simulink model "Cruise_control_V5"  (R2017a)
settings: Solver=VariableStepAuto  StartTime=0.0  StopTime=300  RelTol=1e-3
values from neighbouring files (symbols this model uses):
  DENSITY = 1.164    [parameters.m]
  DRAG_COEFF = 0.2    [parameters.m]
  EMOTOR_EFF = 0.945    [parameters.m]
  energyTotal_noDrag = energyTotal_noDrag/(3600*EMOTOR_EFF)    [parameters.m]
  FRICTION_COEFF = 0.02    [parameters.m]
  HorizontalGravityForce = data(:,4)    [parameters.m]
  MASS = 250    [parameters.m]
  MAX_SPEED = 100/1.60934    (= 62.137273665)    [parameters.m]
  mult_vel_ToPower = mult_vel_ToPower*1.60934/(3.6*EMOTOR_EFF)    [parameters.m]
  mult_velcubed_ToPower = DENSITY*DRAG_COEFF*1.60934^3/(2*3.6^3*EMOTOR_EFF)    (= 0.0110041648249)    [parameters.m]
  mult_velsq_ToDragEnergy = DENSITY*DRAG_COEFF*1000*1.60934^3/(2*3.6^2)    (= 37.4361687342)    [parameters.m]
  NetDistancemiles = data(:,2)    [parameters.m]
  total_distmiles = NetDistancemiles(len)+Distancemiles(len)    [parameters.m]
  WARNING_LIGHT = 0.15    [parameters.m]
undefined symbols (not defined in the file or in its folder): magnitude, sigbuilder_block
libraries: simulink x2, commutil2 x1
settings Model: PauseTimes=15  Creator=marty  LastModifiedBy=marty
settings OptimizationCC: DefaultParameterBehavior=Inlined  UseDivisionForNetSlopeComputation=on  UseFloatMulNetSlope=on  InlineInvariantSignals=on  PassReuseOutputArgsAs=Individual arguments  ZeroExternalMemoryAtStartup=off  ZeroInternalMemoryAtStartup=off  NoFixptDivByZeroProtection=on  EfficientFloat2IntCast=on  LifeSpan=1
settings DebuggingCC: ParameterTunabilityLossMsg=error
settings HardwareCC: ProdBitPerInt=16  ProdBitPerPointer=8  ProdBitPerSizeT=24  ProdBitPerPtrDiffT=24  ProdLargestAtomicFloat=None  ProdWordSize=8  ProdHWDeviceType=Microchip->PIC18
settings SFSimCC: MATLABDynamicMemAlloc=off
settings RTWCC: SystemTargetFile=ert.tlc  TemplateMakefile=ert_default_tmf  Description=Embedded Coder  GenerateReport=on  IncludeHyperlinkInReport=on  LaunchReport=on  GenerateTraceInfo=on  GenerateTraceReport=on  GenerateTraceReportSl=on  GenerateTraceReportSf=on  GenerateTraceReportEml=on  GenerateCodeMetricsReport=on
settings CodeAppCC: ForceParamTrailComments=on  IgnoreCustomStorageClasses=off  OperatorAnnotations=on  SimulinkDataObjDesc=on  SFDataObjDesc=on  MATLABFcnDesc=on  CustomSymbolStrGlobalVar=rt$N$M  CustomSymbolStrType=$N$M  CustomSymbolStrFcn=$N$M$F  CustomSymbolStrMacro=$N$M  InsertBlockDesc=on  MATLABSourceComments=on
settings ERTTargetCC: TargetLangStandard=C99 (ISO)  GenerateSampleERTMain=on  IncludeMdlTerminateFcn=off  CombineSignalStateStructs=on  SupportContinuousTime=on  SupportNonInlinedSFcns=on  SupportVariableSizeSignals=on  InlinedParameterPlacement=NonHierarchical  ERTCustomFileTemplate=example_file_process.tlc  ERTFilePackagingFormat=CompactWithDataFile

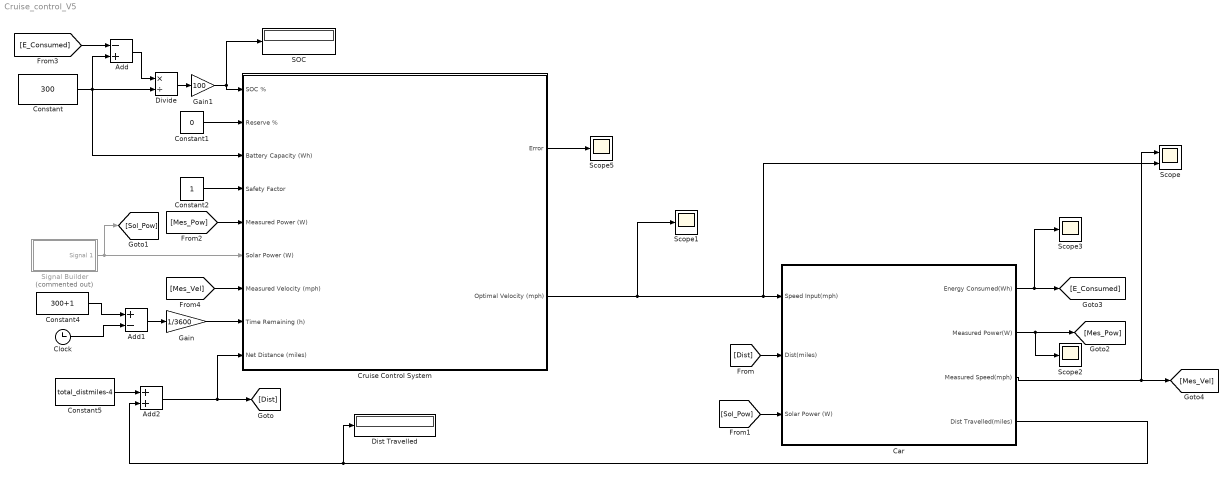
== system Cruise_control_V5 ==
  Add : Sum  Inputs=-+
  Add1 : Sum  Inputs=+-
  Add2 : Sum
  Car : Subsystem
  Clock : Clock
  Constant : Constant  Value=300
  Constant1 : Constant  Value=0
  Constant2 : Constant
  Constant4 : Constant  Value=300+1
  Constant5 : Constant  Value=total_distmiles-4
  Cruise Control System : Subsystem
  Dist Travelled : Display
  Divide : Product  Inputs=*/
  Gain : Gain  Gain=1/3600
  Gain1 : Gain  Gain=100
  SOC : Display
  Scope : Scope  NumInputPorts=2
  Scope{1..3,5} (4 alike) : Scope
  Signal Builder : Subsystem  Tag=STV Subsys  Commented=on  LoadFcn=sigbuilder_block('load');  StartFcn=sigbuilder_block('start');  StopFcn=sigbuilder_block('stop');  ClipboardFcn=sigbuilder_block('clipboard');  mask(Sigbuilder block){tuvar=[0:10]}
      mask help: Simulink:masks:SigbuilderBlock_MD
      mask init:
      | if ~strcmp(get_param(bdroot(gcbh),'SimulationStatus'),'stopped') tuvar = sigbuilder_block('maskInit'); end
      settings: CopyFcn=sigbuilder_block('copy');  DeleteFcn=sigbuilder_block('delete');  ModelCloseFcn=sigbuilder_block('modelClose');  PreSaveFcn=sigbuilder_block('preSave');  PauseFcn=sigbuilder_block('pause');  ContinueFcn=sigbuilder_block('continue');  NameChangeFcn=sigbuilder_block('namechange');  OpenFcn=sigbuilder_block('open',[281.4 73.8 550.8 400.2 ]);  CloseFcn=sigbuilder_block('close');
      mask Display: plot(0, 0, 100, 100,[2, 2, 32, 32, 2], [68, 8, 8, 68, 68],[32, 2], [38, 38], [32, 19, 2],[53, 60, 44], [32, 17, 17, 2],[16, 16, 31, 31]);txt = getActiveGroup(gcbh);text(2, 100, txt,'verticalAlignment', 'top');
  wires:
  Add/1 -> Divide/1
  Constant/1 -> Cruise Control System/3(Battery Capacity (Wh)), Divide/2, Add/2
  Constant1/1 -> Cruise Control System/2(Reserve %)
  Constant2/1 -> Cruise Control System/4(Safety Factor)
  Signal Builder/1(Signal 1) -> [Sol_Pow], Cruise Control System/6(Solar Power (W))
  Constant4/1 -> Add1/1
  Clock/1 -> Add1/2
  Add1/1 -> Gain/1
  Constant5/1 -> Add2/1
  Car/4(Dist Travelled(miles)) -> Dist Travelled/1, Add2/2
  Add2/1 -> [Dist], Cruise Control System/9(Net Distance (miles))
  Divide/1 -> Gain1/1
  Gain1/1 -> SOC/1, Cruise Control System/1(SOC %)
  Gain/1 -> Cruise Control System/8(Time Remaining (h))
  [Dist] -> Car/2(Dist(miles))
  Cruise Control System/1(Error) -> Scope5/1
  [Sol_Pow] -> Car/3(Solar Power (W))
  Car/2(Measured Power(W)) -> Scope2/1, [Mes_Pow]
  [Mes_Pow] -> Cruise Control System/5(Measured Power (W))
  Car/1(Energy Consumed(Wh)) -> Scope3/1, [E_Consumed]
  [E_Consumed] -> Add/1
  Car/3(Measured Speed(mph)) -> Scope/1, [Mes_Vel]
  [Mes_Vel] -> Cruise Control System/7(Measured Velocity (mph))
  Cruise Control System/2(Optimal Velocity (mph)) -> Scope/2, Car/1(Speed Input(mph)), Scope1/1

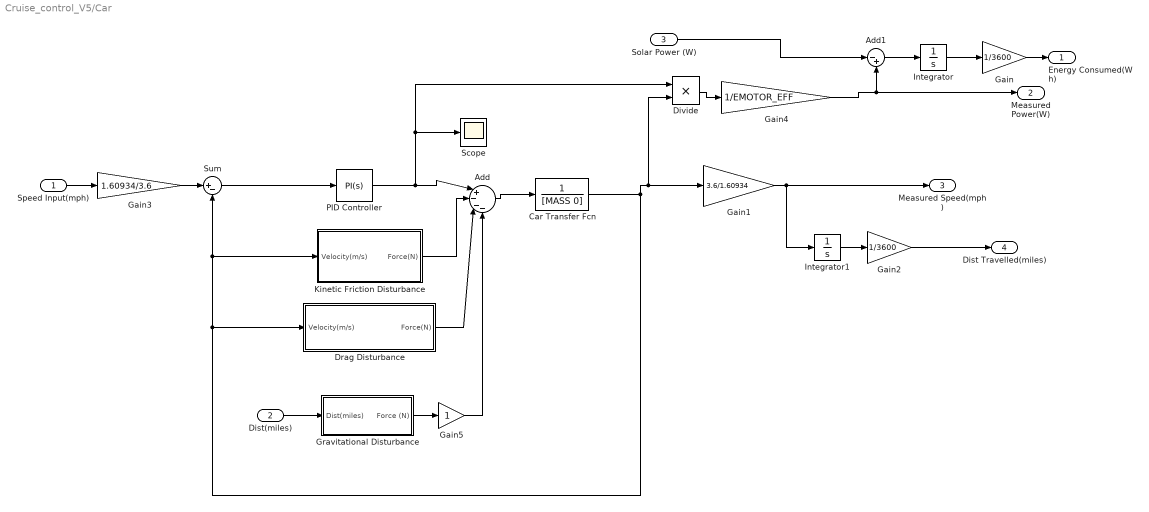
== system Cruise_control_V5/Car ==
  Speed Input(mph) : Inport
  Dist(miles) : Inport  Port=2
  Solar Power (W) : Inport  Port=3
  Add : Sum  Inputs=|+---
  Add1 : Sum  Inputs=|-+
  Car Transfer Fcn : TransferFcn  Denominator=[MASS 0]
  Divide : Product  Inputs=**
  Drag Disturbance : Subsystem
  Gain : Gain  Gain=1/3600
  Gain1 : Gain  Gain=3.6/1.60934
  Gain2 : Gain  Gain=1/3600
  Gain3 : Gain  Gain=1.60934/3.6
  Gain4 : Gain  Gain=1/EMOTOR_EFF
  Gain5 : Gain
  Gravitational Disturbance : Subsystem
  Integrator : Integrator
  Integrator1 : Integrator
  Kinetic Friction Disturbance : Subsystem
  PID Controller : simulink/Continuous/PID Controller  Controller=PI  TimeDomain=Continuous-time  SampleTime=-1  IntegratorMethod=Forward Euler  FilterMethod=Forward Euler  Form=Parallel  UseFilter=on  ControllerParametersSource=internal  P=200  I=19.1491594951774  D=-103.133475492692  N=0.374096308615762  InitialConditionSource=internal  InitialConditionForIntegrator=0  InitialConditionForFilter=0  ExternalReset=none  LimitOutput=off  UpperSaturationLimit=inf  LowerSaturationLimit=-inf  LinearizeAsGain=on  AntiWindupMode=none  Kb=1  TrackingMode=off  Kt=1  PParamMin=[]  PParamMax=[]  IParamMin=[]  IParamMax=[]  DParamMin=[]  DParamMax=[]  NParamMin=[]  NParamMax=[]  KbParamMin=[]  KbParamMax=[]  KtParamMin=[]  KtParamMax=[]  POutMin=[]  POutMax=[]  IOutMin=[]  IOutMax=[]  DOutMin=[]  DOutMax=[]  NOutMin=[]  NOutMax=[]  KbOutMin=[]  KbOutMax=[]  KtOutMin=[]  KtOutMax=[]  IntegratorOutMin=[]  IntegratorOutMax=[]  FilterOutMin=[]  FilterOutMax=[]  SumOutMin=[]  SumOutMax=[]  SumI1OutMin=[]  SumI1OutMax=[]  SumI2OutMin=[]  SumI2OutMax=[]  SumI3OutMin=[]  SumI3OutMax=[]  SumDOutMin=[]  SumDOutMax=[]  SaturationOutMin=[]  SaturationOutMax=[]  IntegratorContinuousStateAttributes=''  IntegratorStateMustResolveToSignalObject=off  IntegratorRTWStateStorageClass=Auto  FilterContinuousStateAttributes=''  FilterStateMustResolveToSignalObject=off  FilterRTWStateStorageClass=Auto  DifferentiatorICPrevScaledInput=0  DifferentiatorOutMin=[]  DifferentiatorOutMax=[]  InitialConditionSetting=State (most efficient)
  Scope : Scope
  Sum : Sum  Inputs=|+-
  Energy Consumed(Wh) : Outport
  Measured Power(W) : Outport  Port=2
  Measured Speed(mph) : Outport  Port=3
  Dist Travelled(miles) : Outport  Port=4
  wires:
  Sum/1 -> PID Controller/1
  Car Transfer Fcn/1 -> Gain1/1, Divide/2, Sum/2, Kinetic Friction Disturbance/1(Velocity(m/s)), Drag Disturbance/1(Velocity(m/s))
  Divide/1 -> Gain4/1
  Integrator/1 -> Gain/1
  Gain/1 -> Energy Consumed(Wh)/1
  Gain3/1 -> Sum/1
  Gain1/1 -> Integrator1/1, Measured Speed(mph)/1
  Integrator1/1 -> Gain2/1
  Gain2/1 -> Dist Travelled(miles)/1
  Speed Input(mph)/1 -> Gain3/1
  Add/1 -> Car Transfer Fcn/1
  Kinetic Friction Disturbance/1(Force(N)) -> Add/2
  Drag Disturbance/1(Force(N)) -> Add/3
  Dist(miles)/1 -> Gravitational Disturbance/1(Dist(miles))
  Gain4/1 -> Add1/2, Measured Power(W)/1
  Add1/1 -> Integrator/1
  Solar Power (W)/1 -> Add1/1
  PID Controller/1 -> Scope/1, Divide/1, Add/1
  Gravitational Disturbance/1(Force (N)) -> Gain5/1
  Gain5/1 -> Add/4

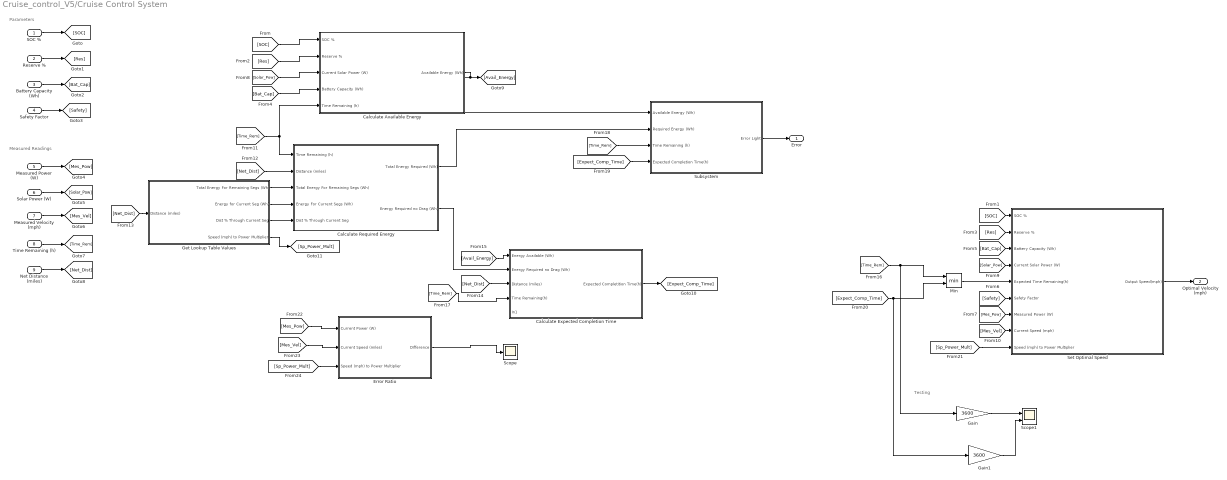
== system Cruise_control_V5/Cruise Control System ==
  note: Testing
  note: Measured Readings
  note: Parameters
  SOC % : Inport
  Reserve % : Inport  Port=2
  Battery Capacity (Wh) : Inport  Port=3
  Safety Factor : Inport  Port=4
  Measured Power (W) : Inport  Port=5
  Solar Power (W) : Inport  Port=6
  Measured Velocity (mph) : Inport  Port=7
  Time Remaining (h) : Inport  Port=8
  Net Distance (miles) : Inport  Port=9
  Calculate Available Energy : Subsystem
  Calculate Expected Completion Time : Subsystem
  Calculate Required Energy : Subsystem
  Error Ratio : Subsystem
  Gain : Gain  Gain=3600
  Gain1 : Gain  Gain=3600
  Get Lookup Table Values : Subsystem
  Min : MinMax  Inputs=2
  Scope : Scope
  Scope1 : Scope  NumInputPorts=2
  Set Optimal Speed : Subsystem
  Subsystem : Subsystem
  Error : Outport
  Optimal Velocity (mph) : Outport  Port=2
  wires:
  Time Remaining (h)/1 -> [Time_Rem]
  Solar Power (W)/1 -> [Solar_Pow]
  Measured Velocity (mph)/1 -> [Mes_Vel]
  [Solar_Pow] -> Set Optimal Speed/4(Current Solar Power (W))
  [Solar_Pow] -> Calculate Available Energy/3(Current Solar Power (W))
  [SOC] -> Set Optimal Speed/1(SOC %)
  Set Optimal Speed/1(Output Speed(mph)) -> Optimal Velocity (mph)/1
  [Res] -> Calculate Available Energy/2(Reserve %)
  Battery Capacity (Wh)/1 -> [Bat_Cap]
  [Bat_Cap] -> Set Optimal Speed/3(Battery Capacity (Wh))
  Net Distance (miles)/1 -> [Net_Dist]
  Get Lookup Table Values/3(Dist % Through Current Seg) -> Calculate Required Energy/5(Dist % Through Current Seg)
  [Mes_Pow] -> Set Optimal Speed/7(Measured Power (W))
  [Bat_Cap] -> Calculate Available Energy/4(Battery Capacity (Wh))
  Measured Power (W)/1 -> [Mes_Pow]
  Get Lookup Table Values/2(Energy for Current Seg (Wh)) -> Calculate Required Energy/4(Energy For Current Segs (Wh))
  Get Lookup Table Values/1(Total Energy For Remaining Segs (Wh)) -> Calculate Required Energy/3(Total Energy For Remaining Segs (Wh))
  [Res] -> Set Optimal Speed/2(Reserve %)
  Reserve %/1 -> [Res]
  [SOC] -> Calculate Available Energy/1(SOC %)
  SOC %/1 -> [SOC]
  [Safety] -> Set Optimal Speed/6(Safety Factor)
  [Net_Dist] -> Calculate Required Energy/2("Distance (miles) ")
  [Mes_Vel] -> Set Optimal Speed/8(Current Speed (mph))
  Safety Factor/1 -> [Safety]
  [Time_Rem] -> Calculate Required Energy/1(Time Remaining (h)), Calculate Available Energy/5(Time Remaining (h))
  Calculate Required Energy/2(Energy Required no Drag (Wh)) -> Calculate Expected Completion Time/2(Energy Required no Drag (Wh))
  [Net_Dist] -> Get Lookup Table Values/1(Distance (miles))
  Calculate Required Energy/1(Total Energy Required (Wh)) -> Subsystem/2(Required Energy (Wh))
  Calculate Available Energy/1(Available Energy (Wh)) -> Subsystem/1(Available Energy (Wh)), [Avail_Energy]
  [Net_Dist] -> Calculate Expected Completion Time/3("Distance (miles) ")
  Min/1 -> Set Optimal Speed/5(Expected Time Remaining(h))
  [Time_Rem] -> Calculate Expected Completion Time/4(Time Remaining(h))
  Gain/1 -> Scope1/1
  Gain1/1 -> Scope1/2
  [Avail_Energy] -> Calculate Expected Completion Time/1(Energy Available (Wh))
  [Time_Rem] -> Min/1, Gain/1
  [Time_Rem] -> Subsystem/3(Time Remaining (h))
  Calculate Expected Completion Time/1("Expected Completition Time(h) ") -> [Expect_Comp_Time]
  [Expect_Comp_Time] -> Subsystem/4(Expected Completion Time(h))
  [Expect_Comp_Time] -> Min/2, Gain1/1
  Get Lookup Table Values/4(Speed (mph) to Power Multiplier) -> [Sp_Power_Mult]
  [Sp_Power_Mult] -> Set Optimal Speed/9(Speed (mph) to Power Multiplier)
  Subsystem/1("Error Light ") -> Error/1
  Error Ratio/1(Difference) -> Scope/1
  [Mes_Pow] -> Error Ratio/1(Current Power (W))
  [Mes_Vel] -> Error Ratio/2(Current Speed (miles))
  [Sp_Power_Mult] -> Error Ratio/3("Speed (mph) to Power Multiplier ")

== system Cruise_control_V5/Signal Builder ==
  Demux : Demux  Tag=STV Demux  Outputs=1
  FromWs : FromWorkspace  Tag=STV FromWs  VariableName=tuvar  SampleTime=0
      SigBuilderData=|
      | common.afterFinalStr = 'Extrapolate'
      | common.sampleTime = 0
      | dataSet.timeRange = [0 120]
      | dataSet.name = 'Group 1'
      | sbobj.Groups.Name = 'Group 1'
      | sbobj.Groups.Signals.Name = 'Signal 1'
      | sbobj.Groups.Signals.XData = [0 4 6 40 40 120]
      | sbobj.Groups.Signals.YData = [0 0 0 0 750 750]
      | sbobj.Groups.TimeRange = [0 120]
  Signal 1 : Outport  Tag=STV Outport
  wires:
  Demux/1 -> Signal 1/1
  FromWs/1 -> Demux/1

== system Cruise_control_V5/Car/Drag Disturbance ==
  Velocity(m/s) : Inport
  Display : Display
  Gain5 : Gain  Gain=DENSITY*DRAG_COEFF/2
  Math Function : Math  Operator=magnitude^2  SaturateOnIntegerOverflow=on
  Force(N) : Outport
  wires:
  Gain5/1 -> Force(N)/1
  Math Function/1 -> Gain5/1
  Velocity(m/s)/1 -> Display/1, Math Function/1

== system Cruise_control_V5/Car/Gravitational Disturbance ==
  Dist(miles) : Inport
  Direct Lookup Table (n-D) : LookupNDDirect  NumberOfTableDimensions=1  Table=[HorizontalGravityForce']
  Prelookup : PreLookup  BreakpointsData=[NetDistancemiles;total_distmiles]
  Force (N) : Outport
  wires:
  Prelookup/1 -> Direct Lookup Table (n-D)/1
  Dist(miles)/1 -> Prelookup/1
  Direct Lookup Table (n-D)/1 -> Force (N)/1

== system Cruise_control_V5/Car/Kinetic Friction Disturbance ==
  Velocity(m/s) : Inport
  Constant : Constant  Value=MASS*9.8*FRICTION_COEFF
  Constant1 : Constant  Value=0
  Switch : Switch  Criteria=u2 > Threshold
  Force(N) : Outport
  wires:
  Switch/1 -> Force(N)/1
  Constant1/1 -> Switch/3
  Velocity(m/s)/1 -> Switch/2
  Constant/1 -> Switch/1

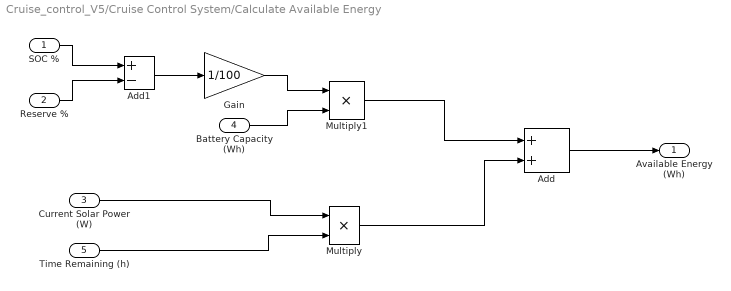
== system Cruise_control_V5/Cruise Control System/Calculate Available Energy ==
  SOC % : Inport
  Reserve % : Inport  Port=2
  Current Solar Power (W) : Inport  Port=3
  Battery Capacity (Wh) : Inport  Port=4
  Time Remaining (h) : Inport  Port=5
  Add : Sum
  Add1 : Sum  Inputs=+-
  Gain : Gain  Gain=1/100
  Multiply : Product  Inputs=**
  Multiply1 : Product  Inputs=**
  Available Energy (Wh) : Outport
  wires:
  SOC %/1 -> Add1/1
  Multiply/1 -> Add/2
  Gain/1 -> Multiply1/1
  Add1/1 -> Gain/1
  Reserve %/1 -> Add1/2
  Multiply1/1 -> Add/1
  Battery Capacity (Wh)/1 -> Multiply1/2
  Current Solar Power (W)/1 -> Multiply/1
  Time Remaining (h)/1 -> Multiply/2
  Add/1 -> Available Energy (Wh)/1

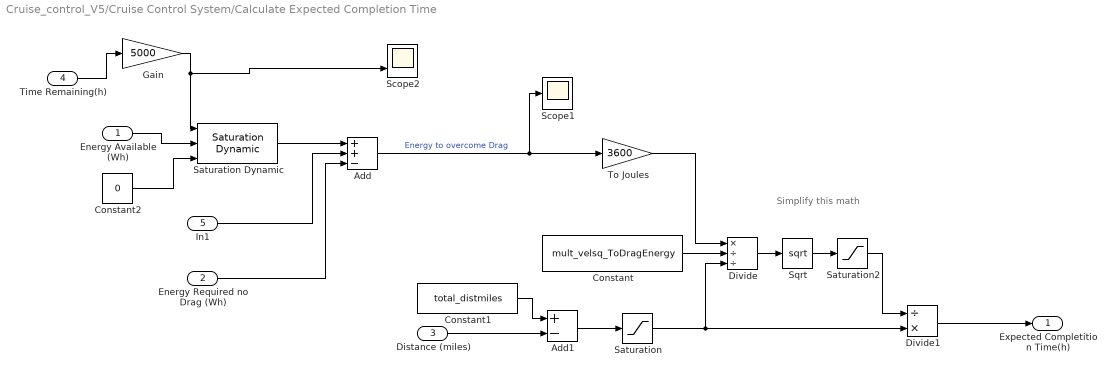
== system Cruise_control_V5/Cruise Control System/Calculate Expected Completion Time ==
  note: Simplify this math
  Energy Available (Wh) : Inport
  Energy Required no Drag (Wh) : Inport  Port=2
  "Distance (miles) " : Inport  Port=3
  Time Remaining(h) : Inport  Port=4
  In1 : Inport  Port=5
  Add : Sum  Inputs=++-
  Add1 : Sum  Inputs=+-
  Constant : Constant  Value=mult_velsq_ToDragEnergy  SampleTime=-1
  Constant1 : Constant  Value=total_distmiles
  Constant2 : Constant  Value=0
  Divide : Product  Inputs=*//
  Divide1 : Product  Inputs=/*
  Gain : Gain  Gain=5000
  Saturation : Saturate  UpperLimit=inf  LowerLimit=0
  Saturation Dynamic : simulink/Discontinuities/Saturation Dynamic  OutMin=[]  OutMax=[]  OutDataTypeStr=Inherit: Same as second input  OutDataType=fixdt(1, 16)  OutScaling=2^-10  DoSatur=off
  Saturation2 : Saturate  UpperLimit=MAX_SPEED  LowerLimit=0
  Scope1 : Scope
  Scope2 : Scope  NumInputPorts=2
  Sqrt : Sqrt  SaturateOnIntegerOverflow=on
  To Joules : Gain  Gain=3600
  "Expected Completition Time(h) " : Outport
  wires:
  Add/1 -> Scope1/1, To Joules/1  "Energy to overcome Drag"
  To Joules/1 -> Divide/1
  Sqrt/1 -> Saturation2/1
  Divide1/1 -> "Expected Completition Time(h) "/1
  Constant1/1 -> Add1/1
  "Distance (miles) "/1 -> Add1/2
  Constant/1 -> Divide/2
  Add1/1 -> Saturation/1
  Saturation/1 -> Divide1/2, Divide/3
  Time Remaining(h)/1 -> Gain/1
  Constant2/1 -> Saturation Dynamic/3
  Gain/1 -> Saturation Dynamic/1, Scope2/2
  Saturation Dynamic/1 -> Add/1
  Energy Available (Wh)/1 -> Saturation Dynamic/2
  Divide/1 -> Sqrt/1
  Saturation2/1 -> Divide1/1
  In1/1 -> Add/2
  Energy Required no Drag (Wh)/1 -> Add/3

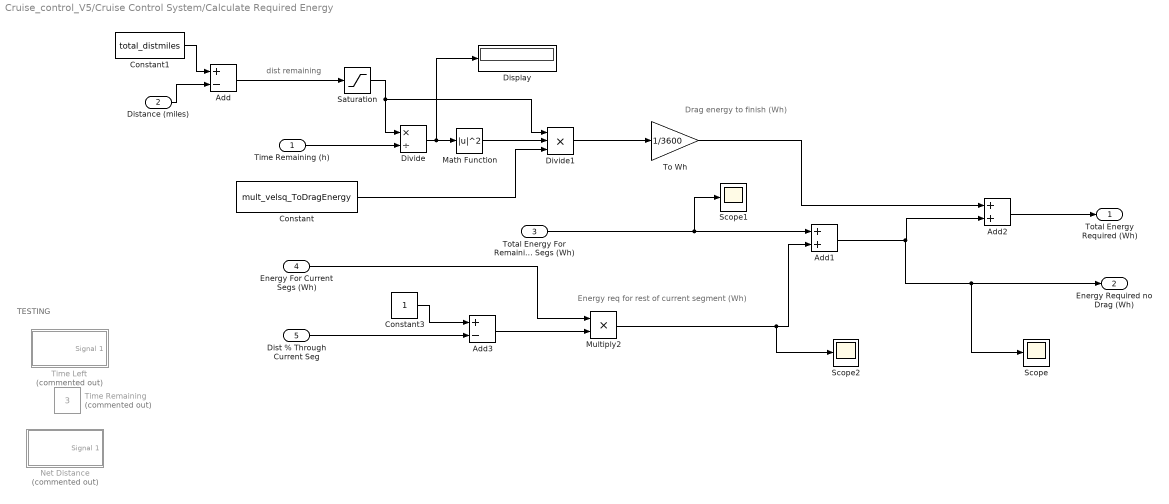
== system Cruise_control_V5/Cruise Control System/Calculate Required Energy ==
  note: TESTING
  note: Drag energy to finish (Wh)
  note: dist remaining
  note: Energy req for rest of current segment (Wh)
  Time Remaining (h) : Inport
  "Distance (miles) " : Inport  Port=2
  Total Energy For Remaining Segs (Wh) : Inport  Port=3
  Energy For Current Segs (Wh) : Inport  Port=4
  Dist % Through Current Seg : Inport  Port=5
  Add : Sum  Inputs=+-
  Add1 : Sum
  Add2 : Sum
  Add3 : Sum  Inputs=+-
  Constant : Constant  Value=mult_velsq_ToDragEnergy  SampleTime=-1
  Constant1 : Constant  Value=total_distmiles
  Constant3 : Constant
  Display : Display
  Divide : Product  Inputs=*/
  Divide1 : Product  Inputs=***
  Math Function : Math  Operator=magnitude^2  SaturateOnIntegerOverflow=on
  Multiply2 : Product  Inputs=**
  Net Distance : Subsystem  Tag=STV Subsys  Commented=on  LoadFcn=sigbuilder_block('load');  StartFcn=sigbuilder_block('start');  StopFcn=sigbuilder_block('stop');  ClipboardFcn=sigbuilder_block('clipboard');  mask(Sigbuilder block){tuvar=[0:10]}
      mask help: Simulink:masks:SigbuilderBlock_MD
      mask init:
      | if ~strcmp(get_param(bdroot(gcbh),'SimulationStatus'),'stopped') tuvar = sigbuilder_block('maskInit'); end
      settings: CopyFcn=sigbuilder_block('copy');  DeleteFcn=sigbuilder_block('delete');  ModelCloseFcn=sigbuilder_block('modelClose');  PreSaveFcn=sigbuilder_block('preSave');  PauseFcn=sigbuilder_block('pause');  ContinueFcn=sigbuilder_block('continue');  NameChangeFcn=sigbuilder_block('namechange');  OpenFcn=sigbuilder_block('open',[323.4 109.8 550.8 400.2 ]);  CloseFcn=sigbuilder_block('close');
      mask Display: plot(0, 0, 100, 100,[2, 2, 32, 32, 2], [68, 8, 8, 68, 68],[32, 2], [38, 38], [32, 19, 2],[53, 60, 44], [32, 17, 17, 2],[16, 16, 31, 31]);txt = getActiveGroup(gcbh);text(2, 100, txt,'verticalAlignment', 'top');
  Saturation : Saturate  UpperLimit=inf  LowerLimit=0
  Scope : Scope
  Scope1 : Scope
  Scope2 : Scope
  Time Left : Subsystem  Tag=STV Subsys  Commented=on  LoadFcn=sigbuilder_block('load');  StartFcn=sigbuilder_block('start');  StopFcn=sigbuilder_block('stop');  ClipboardFcn=sigbuilder_block('clipboard');  mask(Sigbuilder block){tuvar=[0:10]}
      mask help: Simulink:masks:SigbuilderBlock_MD
      mask init:
      | if ~strcmp(get_param(bdroot(gcbh),'SimulationStatus'),'stopped') tuvar = sigbuilder_block('maskInit'); end
      settings: CopyFcn=sigbuilder_block('copy');  DeleteFcn=sigbuilder_block('delete');  ModelCloseFcn=sigbuilder_block('modelClose');  PreSaveFcn=sigbuilder_block('preSave');  PauseFcn=sigbuilder_block('pause');  ContinueFcn=sigbuilder_block('continue');  NameChangeFcn=sigbuilder_block('namechange');  OpenFcn=sigbuilder_block('open',[323.4 109.8 550.8 400.2 ]);  CloseFcn=sigbuilder_block('close');
      mask Display: plot(0, 0, 100, 100,[2, 2, 32, 32, 2], [68, 8, 8, 68, 68],[32, 2], [38, 38], [32, 19, 2],[53, 60, 44], [32, 17, 17, 2],[16, 16, 31, 31]);txt = getActiveGroup(gcbh);text(2, 100, txt,'verticalAlignment', 'top');
  Time Remaining : Constant  Commented=on  Value=3
  To Wh : Gain  Gain=1/3600
  Total Energy Required (Wh) : Outport
  Energy Required no Drag (Wh) : Outport  Port=2
  wires:
  Divide1/1 -> To Wh/1
  Constant1/1 -> Add/1
  To Wh/1 -> Add2/1
  "Distance (miles) "/1 -> Add/2
  Add2/1 -> Total Energy Required (Wh)/1
  Total Energy For Remaining Segs (Wh)/1 -> Scope1/1, Add1/1
  Energy For Current Segs (Wh)/1 -> Multiply2/1
  Dist % Through Current Seg/1 -> Add3/2
  Multiply2/1 -> Scope2/1, Add1/2
  Add3/1 -> Multiply2/2
  Constant3/1 -> Add3/1
  Time Remaining (h)/1 -> Divide/2
  Add/1 -> Saturation/1
  Divide/1 -> Display/1, Math Function/1
  Math Function/1 -> Divide1/2
  Constant/1 -> Divide1/3
  Saturation/1 -> Divide1/1, Divide/1
  Add1/1 -> Scope/1, Energy Required no Drag (Wh)/1, Add2/2

== system Cruise_control_V5/Cruise Control System/Error Ratio ==
  Current Power (W) : Inport
  Current Speed (miles) : Inport  Port=2
  "Speed (mph) to Power Multiplier " : Inport  Port=3
  Add : Sum  Inputs=-+
  Scope : Scope  NumInputPorts=2
  Speed to Expected Power : Subsystem
  Difference : Outport
  wires:
  Current Speed (miles)/1 -> Speed to Expected Power/1(Current Speed (miles))
  Current Power (W)/1 -> Scope/2, Add/1
  Speed to Expected Power/1(Expected Power (W)) -> Scope/1, Add/2
  Add/1 -> Difference/1
  "Speed (mph) to Power Multiplier "/1 -> Speed to Expected Power/2(Speed (mph) to Power Multiplier)

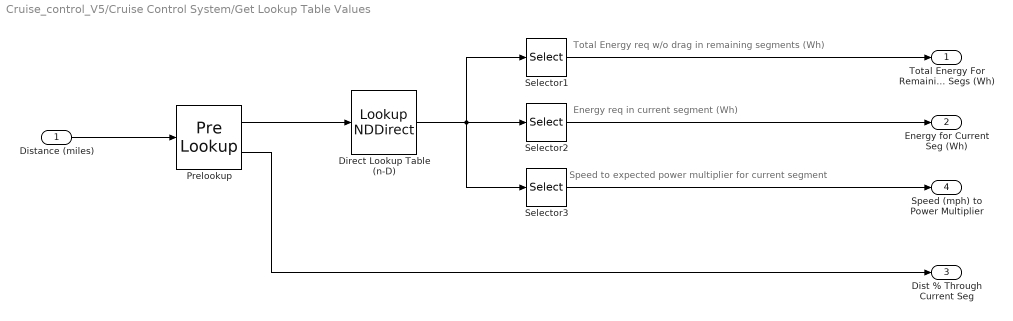
== system Cruise_control_V5/Cruise Control System/Get Lookup Table Values ==
  note: Speed to expected power multiplier for current segment
  note: Energy req in current segment (Wh)
  note: Total Energy req w/o drag in remaining segments (Wh)
  Distance (miles) : Inport
  Direct Lookup Table (n-D) : LookupNDDirect  InputsSelectThisObjectFromTable=Column  Table=[energyTotal_noDrag';energySeg_noDrag';mult_vel_ToPower']
  Prelookup : PreLookup  BreakpointsData=[NetDistancemiles;total_distmiles]
  Selector1 : Selector  InputPortWidth=3  IndexOptions=Index vector (dialog)  Indices=1  OutputSizes=1
  Selector2 : Selector  InputPortWidth=3  IndexOptions=Index vector (dialog)  Indices=2  OutputSizes=1
  Selector3 : Selector  InputPortWidth=3  IndexOptions=Index vector (dialog)  Indices=3  OutputSizes=1
  Total Energy For Remaining Segs (Wh) : Outport
  Energy for Current Seg (Wh) : Outport  Port=2
  Dist % Through Current Seg : Outport  Port=3
  Speed (mph) to Power Multiplier : Outport  Port=4
  wires:
  Direct Lookup Table (n-D)/1 -> Selector3/1, Selector1/1, Selector2/1
  Selector2/1 -> Energy for Current Seg (Wh)/1
  Prelookup/1 -> Direct Lookup Table (n-D)/1
  Prelookup/2 -> Dist % Through Current Seg/1
  Selector1/1 -> Total Energy For Remaining Segs (Wh)/1
  Selector3/1 -> Speed (mph) to Power Multiplier/1
  Distance (miles)/1 -> Prelookup/1

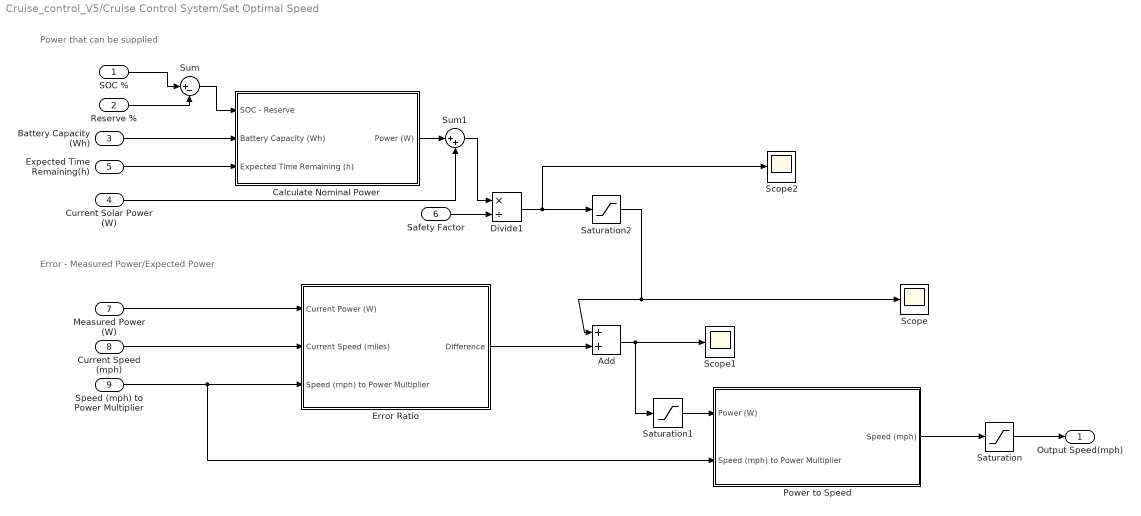
== system Cruise_control_V5/Cruise Control System/Set Optimal Speed ==
  note: Error - Measured Power/Expected Power
  note: Power that can be supplied
  SOC % : Inport
  Reserve % : Inport  Port=2
  Battery Capacity (Wh) : Inport  Port=3
  Current Solar Power (W) : Inport  Port=4
  Expected Time Remaining(h) : Inport  Port=5
  Safety Factor : Inport  Port=6
  Measured Power (W) : Inport  Port=7
  Current Speed (mph) : Inport  Port=8
  Speed (mph) to Power Multiplier : Inport  Port=9
  Add : Sum
  Calculate Nominal Power : Subsystem
  Divide1 : Product  Inputs=*/
  Error Ratio : Subsystem
  Power to Speed : Subsystem
  Saturation : Saturate  UpperLimit=MAX_SPEED  LowerLimit=0
  Saturation1 : Saturate  UpperLimit=inf  LowerLimit=0
  Saturation2 : Saturate  UpperLimit=5000  LowerLimit=0
  Scope : Scope
  Scope1 : Scope
  Scope2 : Scope
  Sum : Sum  Inputs=|+-
  Sum1 : Sum  Inputs=|++
  Output Speed(mph) : Outport
  wires:
  Sum/1 -> Calculate Nominal Power/1(SOC - Reserve)
  SOC %/1 -> Sum/1
  Safety Factor/1 -> Divide1/2
  Calculate Nominal Power/1(Power (W)) -> Sum1/1
  Current Solar Power (W)/1 -> Sum1/2
  Sum1/1 -> Divide1/1
  Reserve %/1 -> Sum/2
  Battery Capacity (Wh)/1 -> Calculate Nominal Power/2(Battery Capacity (Wh))
  Measured Power (W)/1 -> Error Ratio/1(Current Power (W))
  Current Speed (mph)/1 -> Error Ratio/2(Current Speed (miles))
  Power to Speed/1(Speed (mph)) -> Saturation/1
  Saturation/1 -> Output Speed(mph)/1
  Divide1/1 -> Scope2/1, Saturation2/1
  Speed (mph) to Power Multiplier/1 -> Power to Speed/2(Speed (mph) to Power Multiplier), Error Ratio/3("Speed (mph) to Power Multiplier ")
  Saturation1/1 -> Power to Speed/1(Power (W))
  Expected Time Remaining(h)/1 -> Calculate Nominal Power/3(Expected Time Remaining (h))
  Add/1 -> Saturation1/1, Scope1/1
  Error Ratio/1(Difference) -> Add/2
  Saturation2/1 -> Add/1, Scope/1

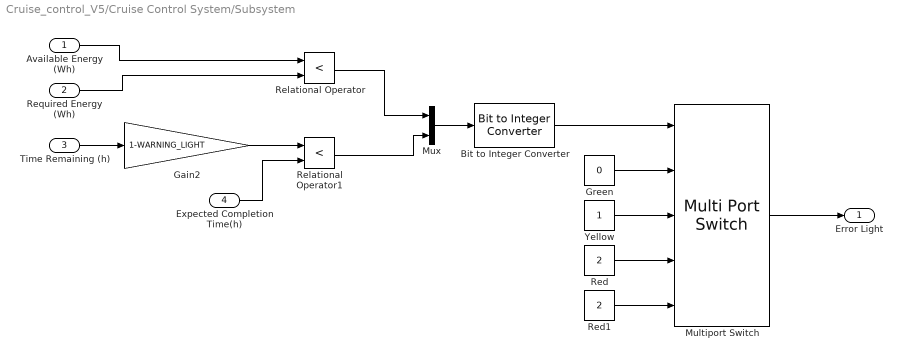
== system Cruise_control_V5/Cruise Control System/Subsystem ==
  Available Energy (Wh) : Inport
  Required Energy (Wh) : Inport  Port=2
  Time Remaining (h) : Inport  Port=3
  Expected Completion Time(h) : Inport  Port=4
  Bit to Integer Converter : commutil2/Bit to Integer Converter  nbits=2  bitOrder=MSB first  signedOutputValues=Unsigned  outDtype=Inherit via internal rule  outDtypeSigned=Inherit via internal rule
  Gain2 : Gain  Gain=1-WARNING_LIGHT
  Green : Constant  Value=0
  Multiport Switch : MultiPortSwitch  DataPortOrder=Zero-based contiguous  Inputs=4  DiagnosticForDefault=None
  Mux : Mux  Inputs=2
  Red : Constant  Value=2
  Red1 : Constant  Value=2
  Relational Operator : RelationalOperator  Operator=<  OutDataTypeStr=boolean  RndMeth=Nearest
  Relational Operator1 : RelationalOperator  Operator=<  OutDataTypeStr=boolean  RndMeth=Simplest
  Yellow : Constant
  "Error Light " : Outport
  wires:
  Gain2/1 -> Relational Operator1/1
  Yellow/1 -> Multiport Switch/3
  Expected Completion Time(h)/1 -> Relational Operator1/2
  Bit to Integer Converter/1 -> Multiport Switch/1
  Red1/1 -> Multiport Switch/5
  Green/1 -> Multiport Switch/2
  Red/1 -> Multiport Switch/4
  Relational Operator1/1 -> Mux/2
  Time Remaining (h)/1 -> Gain2/1
  Mux/1 -> Bit to Integer Converter/1
  Available Energy (Wh)/1 -> Relational Operator/1
  Required Energy (Wh)/1 -> Relational Operator/2
  Relational Operator/1 -> Mux/1
  Multiport Switch/1 -> "Error Light "/1

== system Cruise_control_V5/Cruise Control System/Calculate Required Energy/Net Distance ==
  Demux : Demux  Tag=STV Demux  Outputs=1
  FromWs : FromWorkspace  Tag=STV FromWs  VariableName=tuvar  SampleTime=0
      SigBuilderData=|
      | common.afterFinalStr = 'Extrapolate'
      | common.sampleTime = 0
      | dataSet.timeRange = [0 120]
      | dataSet.name = 'Group 1'
      | sbobj.Groups.Name = 'Group 1'
      | sbobj.Groups.Signals.Name = 'Signal 1'
      | sbobj.Groups.Signals.XData = [0 10 110 120]
      | sbobj.Groups.Signals.YData = [0 0 1985 1985]
      | sbobj.Groups.TimeRange = [0 120]
  Signal 1 : Outport  Tag=STV Outport
  wires:
  Demux/1 -> Signal 1/1
  FromWs/1 -> Demux/1

== system Cruise_control_V5/Cruise Control System/Calculate Required Energy/Time Left ==
  Demux : Demux  Tag=STV Demux  Outputs=1
  FromWs : FromWorkspace  Tag=STV FromWs  VariableName=tuvar  SampleTime=0
      SigBuilderData=|
      | common.afterFinalStr = 'Extrapolate'
      | common.sampleTime = 0
      | dataSet.timeRange = [0 120]
      | dataSet.name = 'Group 1'
      | sbobj.Groups.Name = 'Group 1'
      | sbobj.Groups.Signals.Name = 'Signal 1'
      | sbobj.Groups.Signals.XData = [0 10 110 120]
      | sbobj.Groups.Signals.YData = [100 100 1 1]
      | sbobj.Groups.TimeRange = [0 120]
  Signal 1 : Outport  Tag=STV Outport
  wires:
  Demux/1 -> Signal 1/1
  FromWs/1 -> Demux/1

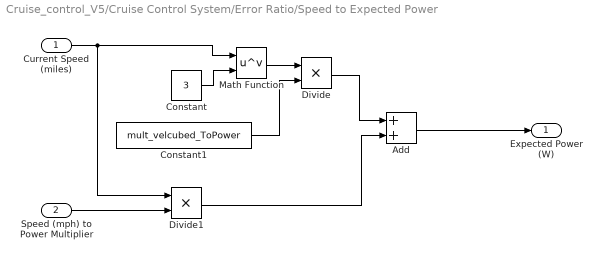
== system Cruise_control_V5/Cruise Control System/Error Ratio/Speed to Expected Power ==
  Current Speed (miles) : Inport
  Speed (mph) to Power Multiplier : Inport  Port=2
  Add : Sum
  Constant : Constant  Value=3
  Constant1 : Constant  Value=mult_velcubed_ToPower
  Divide : Product  Inputs=**
  Divide1 : Product  Inputs=**
  Math Function : Math  Operator=pow  SaturateOnIntegerOverflow=on
  Expected Power (W) : Outport
  wires:
  Constant/1 -> Math Function/2
  Math Function/1 -> Divide/1
  Constant1/1 -> Divide/2
  Current Speed (miles)/1 -> Divide1/1, Math Function/1
  Speed (mph) to Power Multiplier/1 -> Divide1/2
  Add/1 -> Expected Power (W)/1
  Divide/1 -> Add/1
  Divide1/1 -> Add/2

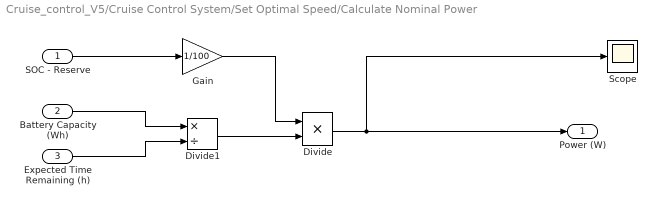
== system Cruise_control_V5/Cruise Control System/Set Optimal Speed/Calculate Nominal Power ==
  SOC - Reserve : Inport
  Battery Capacity (Wh) : Inport  Port=2
  Expected Time Remaining (h) : Inport  Port=3
  Divide : Product  Inputs=**
  Divide1 : Product  Inputs=*/
  Gain : Gain  Gain=1/100
  Scope : Scope
  Power (W) : Outport
  wires:
  SOC - Reserve/1 -> Gain/1
  Gain/1 -> Divide/1
  Battery Capacity (Wh)/1 -> Divide1/1
  Divide1/1 -> Divide/2
  Expected Time Remaining (h)/1 -> Divide1/2
  Divide/1 -> Power (W)/1, Scope/1

== system Cruise_control_V5/Cruise Control System/Set Optimal Speed/Error Ratio ==
  Current Power (W) : Inport
  Current Speed (miles) : Inport  Port=2
  "Speed (mph) to Power Multiplier " : Inport  Port=3
  Add : Sum  Inputs=-+
  Scope : Scope  NumInputPorts=2
  Speed to Expected Power : Subsystem
  Difference : Outport
  wires:
  Current Speed (miles)/1 -> Speed to Expected Power/1(Current Speed (miles))
  Current Power (W)/1 -> Scope/2, Add/1
  Speed to Expected Power/1(Expected Power (W)) -> Scope/1, Add/2
  Add/1 -> Difference/1
  "Speed (mph) to Power Multiplier "/1 -> Speed to Expected Power/2(Speed (mph) to Power Multiplier)

== system Cruise_control_V5/Cruise Control System/Set Optimal Speed/Power to Speed ==
  Power (W) : Inport
  Speed (mph) to Power Multiplier : Inport  Port=2
  MATLAB Function : MATLAB Function  TreatAsAtomicUnit=on
  Speed (mph) : Outport
  wires:
  MATLAB Function/1(speed_mph) -> Speed (mph)/1
  Speed (mph) to Power Multiplier/1 -> MATLAB Function/2(vel_to_power_mult)
  Power (W)/1 -> MATLAB Function/1(power)

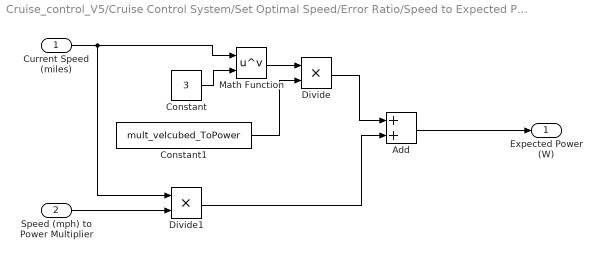
== system Cruise_control_V5/Cruise Control System/Set Optimal Speed/Error Ratio/Speed to Expected Power ==
  Current Speed (miles) : Inport
  Speed (mph) to Power Multiplier : Inport  Port=2
  Add : Sum
  Constant : Constant  Value=3
  Constant1 : Constant  Value=mult_velcubed_ToPower
  Divide : Product  Inputs=**
  Divide1 : Product  Inputs=**
  Math Function : Math  Operator=pow  SaturateOnIntegerOverflow=on
  Expected Power (W) : Outport
  wires:
  Constant/1 -> Math Function/2
  Math Function/1 -> Divide/1
  Constant1/1 -> Divide/2
  Current Speed (miles)/1 -> Divide1/1, Math Function/1
  Speed (mph) to Power Multiplier/1 -> Divide1/2
  Add/1 -> Expected Power (W)/1
  Divide/1 -> Add/1
  Divide1/1 -> Add/2

== matlab function Cruise_control_V5/Cruise Control System/Set Optimal Speed/Power to Speed/MATLAB Function ==
  data: speed_mph output; power input double; mult_velcubed_ToPower parameter; vel_to_power_mult input
function speed_mph = fcn(power,mult_velcubed_ToPower, vel_to_power_mult)

r=ones(3,2);
r=roots([mult_velcubed_ToPower 0 vel_to_power_mult -power]);

r=r(abs(imag(r))<1e-5);

if(isempty(r))
    speed_mph=-10;%change this 
else
speed_mph = real(r(1));
end
